simulink model "RPL_3D_Mode_BlocksetApproach"  (R2021b)
settings: Solver=VariableStepAuto  StartTime=0.0  StopTime=10.0  RelTol=1e-3
values from neighbouring files (symbols this model uses):
  Ar = pi*R_rad^2    (= 0.00282743338823)    [constants1DoF.m]
  Cd = 0.5    [constants1DoF.m]
  g = 9.81    [constants1DoF.m]
  m_d_c = 0.01    [constants1DoF.m]
  m_r = 0.5    [constants1DoF.m]
  rho = 1.225    [constants1DoF.m]
  t_burn = 2    [constants1DoF.m]
  Tmax = 10    [constants1DoF.m]
libraries: aerolibbdyn x2, sharedutil x1, aerolibanim x1, aerolib6dof2 x1
settings Model: Creator=josep  LastModifiedBy=josepfamador

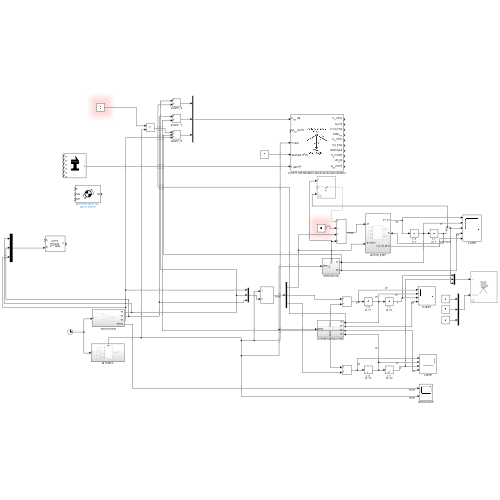
[thumbnail: Simulink's stored preview of the top-level diagram]
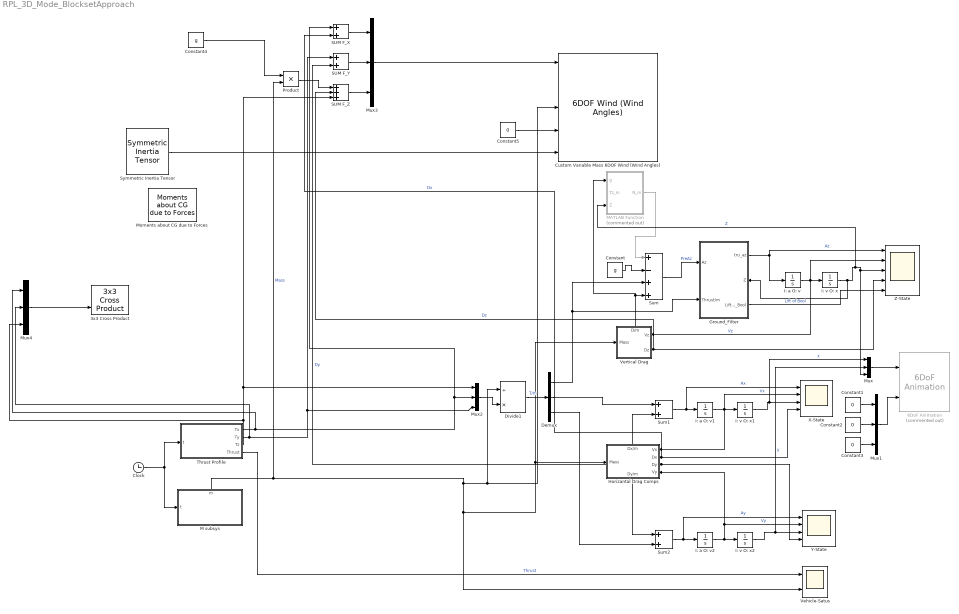
== system RPL_3D_Mode_BlocksetApproach ==
  3x3 Cross Product : sharedutil/3x3 Cross Product  aMode=aMode
      settings: SourceProductBaseCode=AE,PW,DR,MT,UV,VE
  6DoF Animation : aerolibanim/6DoF Animation  Commented=on  u1=[-400 400 -200 200 -500 -300]  u2=0.1  u3=10.0  u4=[0 0 0]  u5=Cockpit  u6=[100 50 -50]  u7=10  u8=on
  Clock : Clock
      settings: Decimation=5
  Constant : Constant  Value=g
  Constant{1..3,5} (4 alike) : Constant  Value=0
  Constant4 : Constant  Value=g
  Custom Variable Mass 6DOF Wind (Wind Angles) : aerolib6dof2/6DOF Wind (Wind Angles)  units=Metric (MKS)  mtype=Custom Variable  rep=Wind Angles  xme_0=[0 0 0]  Vm_0=[0 0 0]  wind_0=[0 0 0]  pm_0=[0 0 0]  mass_0=1.0  mass_e=0.5  mass_f=2.0  inertia=eye(3)  inertia_e=eye(3)  inertia_f=2*eye(3)  vre_flag=off  abi_flag=off  xme_statename=''  Vm_statename=''  alpha_statename=''  beta_statename=''  wind_statename=''  quat_statename=''  pm_statename=''  mass_statename=''
      settings: SourceProductBaseCode=AE
  Demux : Demux  Outputs=3
  Divide1 : Product  Inputs=/*
  Ground_Filter : Subsystem
      settings: PortSchema="{\"entries\":[{\"content\":{\"sides\":[{\"content\":{\"connectorIds\":[\"In1\",\"In2\"]},\"type\":\"ConnectorPlacement.EquallySpacedRectSide\",\"uuid\":\"02f139e3-c71d-4215-a05c-2ea7cb935f0c\"},{\"content\":{\"connectorIds\":[\"Out1\",\"In3\",\"Out2\"],\"side\":\"RIGHT\"},\"type\":\"ConnectorPlacement.EquallySpacedRectSide\",\"uuid\":\"f8d88dc7-1706-414e-8763-66b2344e60f3\"},{\"content\":{\"connectorIds\":[],\"side\":\"TOP\"},\"type\":\"ConnectorPlacement.EquallySpacedRectSide\",\"uuid\":\"2e6fab3d-690f-4ad2-8e7d-0c65fcb07007\"}]},\"type\":\"ConnectorPlacement.EquallySpacedConnector\",\"uuid\":\"04f6aaf0-68c8-473c-8854-b1e33576e060\"}],\"packageUris\":[\"http://schema.mathworks.com/mf0/Connector/R2020b\"],\"version\":\"1.0\"}"
  Horizantal Drag Comps : Subsystem
      settings: PortSchema="{\"entries\":[{\"content\":{\"sides\":[{\"content\":{\"connectorIds\":[\"In1\"]},\"type\":\"ConnectorPlacement.EquallySpacedRectSide\",\"uuid\":\"a9ae7cae-0740-4af7-9b70-c16e835fd7b3\"},{\"content\":{\"connectorIds\":[\"In2\",\"Out1\",\"Out2\",\"In3\"],\"side\":\"RIGHT\"},\"type\":\"ConnectorPlacement.EquallySpacedRectSide\",\"uuid\":\"8697e8bb-b6ea-43ee-b298-40652abd00a9\"},{\"content\":{\"connectorIds\":[\"Out4\"],\"side\":\"TOP\"},\"type\":\"ConnectorPlacement.EquallySpacedRectSide\",\"uuid\":\"6019ad8c-fb7f-40d5-87eb-98a170a5ecc9\"},{\"content\":{\"connectorIds\":[\"Out3\"],\"side\":\"BOTTOM\"},\"type\":\"ConnectorPlacement.EquallySpacedRectSide\",\"uuid\":\"b4d29286-deca-444a-b294-c191927f4c5c\"}]},\"type\":\"ConnectorPlacement.EquallySpacedConnector\",\"uuid\":\"482fa5f4-cfef-448e-9d08-7fbc847693c8\"}],\"packageUris\":[\"http://schema.mathworks.com/mf0/Connector/R2020b\"],\"version\":\"1.0\"}"
  I: a O: v : Integrator
  I: a O: v1 : Integrator
  I: a O: v2 : Integrator
  I: v O: x : Integrator  LowerSaturationLimit=0
  I: v O: x1 : Integrator  LowerSaturationLimit=0
  I: v O: x2 : Integrator  LowerSaturationLimit=0
  M subsys : Subsystem
      settings: PortSchema="{\"entries\":[{\"content\":{\"sides\":[{\"content\":{\"connectorIds\":[\"In1\"]},\"type\":\"ConnectorPlacement.EquallySpacedRectSide\",\"uuid\":\"59fe94dd-ab30-4deb-857c-de4b730c9c49\"},{\"content\":{\"connectorIds\":[],\"side\":\"RIGHT\"},\"type\":\"ConnectorPlacement.EquallySpacedRectSide\",\"uuid\":\"6db86113-106d-42a4-8531-3673608ca4b9\"},{\"content\":{\"connectorIds\":[\"Out1\"],\"side\":\"TOP\"},\"type\":\"ConnectorPlacement.EquallySpacedRectSide\",\"uuid\":\"45854090-be75-4cdf-9468-5c433929868a\"}]},\"type\":\"ConnectorPlacement.EquallySpacedConnector\",\"uuid\":\"b924312b-0fe7-4021-be64-7e2ca8cc4ab7\"}],\"packageUris\":[\"http://schema.mathworks.com/mf0/Connector/R2020b\"],\"version\":\"1.0\"}"
  MATLAB Function : MATLAB Function  Commented=on  TreatAsAtomicUnit=on
  Moments about CG due to Forces : aerolibbdyn/Moments about CG  due to Forces
      settings: SourceProductBaseCode=AE
  Mux{,1..4} (5 alike) : Mux  Inputs=3
  Product : Product
  SUM F_X : Sum
  SUM F_Y : Sum
  SUM F_Z : Sum  Inputs=+++
  Sum : Sum  Inputs=+-++
  Sum1 : Sum
  Sum2 : Sum
  Symmetric Inertia Tensor : aerolibbdyn/Symmetric Inertia Tensor
      settings: SourceProductBaseCode=AE
  Thrust Profile : Subsystem
  Vehicle-Satus : Scope  NumInputPorts=2
  Vertical Drag : Subsystem
      settings: PortSchema="{\"entries\":[{\"content\":{\"sides\":[{\"content\":{\"connectorIds\":[\"In1\"]},\"type\":\"ConnectorPlacement.EquallySpacedRectSide\",\"uuid\":\"72cb64b5-de92-49f0-81ee-1566d770d166\"},{\"content\":{\"connectorIds\":[\"In2\",\"Out1\"],\"side\":\"RIGHT\"},\"type\":\"ConnectorPlacement.EquallySpacedRectSide\",\"uuid\":\"ba77af52-770b-4a76-8b2e-e7cb196d7331\"},{\"content\":{\"connectorIds\":[\"Out2\"],\"side\":\"TOP\"},\"type\":\"ConnectorPlacement.EquallySpacedRectSide\",\"uuid\":\"b46aeb0c-d0a3-4548-b994-998d7dcb34ee\"}]},\"type\":\"ConnectorPlacement.EquallySpacedConnector\",\"uuid\":\"4a9965ec-71ae-4d95-8721-5a5c59972a5c\"}],\"packageUris\":[\"http://schema.mathworks.com/mf0/Connector/R2020b\"],\"version\":\"1.0\"}"
  X-State : Scope  NumInputPorts=4
  Y-State : Scope  NumInputPorts=4
  Z-State : Scope  NumInputPorts=5
  wires:
  Horizantal Drag Comps/4(Dx/m) -> Sum1/2
  Thrust Profile/1(Tx) -> Mux4/1, Mux2/2, SUM F_X/1
  Ground_Filter/2(Lift_off_Bool) -> Z-State/5  "Lift of Bool"
  Vertical Drag/2(D/m) -> MATLAB Function/1(g), Sum/4
  MATLAB Function/1(N_m) -> Sum/1
  Sum/1 -> Ground_Filter/1(Az)  "PreAz"
  Horizantal Drag Comps/2(Dy) -> Y-State/4, SUM F_Y/2  "Dy"
  Sum1/1 -> X-State/1, I: a O: v1/1  "Ax"
  Thrust Profile/2(Ty) -> Mux4/2, SUM F_Y/1, Mux2/3
  Vertical Drag/1(Dz) -> Z-State/4, SUM F_Z/2  "Dz"
  M subsys/1(m) -> Custom Variable Mass 6DOF Wind (Wind Angles)/3, Divide1/1, Vehicle-Satus/2, Vertical Drag/1(Mass), Horizantal Drag Comps/1(Mass), Product/2  "Mass"
  Thrust Profile/3(Tz) -> Mux4/3, SUM F_Z/3, Mux2/1
  Horizantal Drag Comps/1(Dx) -> X-State/4, SUM F_X/2  "Dx"
  Constant3/1 -> Mux1/3
  Ground_Filter/1(tru_az) -> I: a O: v/1, Z-State/1  "Az"
  Constant/1 -> Sum/2
  Constant1/1 -> Mux1/1
  I: a O: v/1 -> Vertical Drag/2(Vz), Z-State/2, I: v O: x/1  "Vz"
  Mux/1 -> 6DoF Animation/1
  Constant2/1 -> Mux1/2
  I: v O: x/1 -> Ground_Filter/3(Z), MATLAB Function/3(Z), Mux/3, Z-State/3  "Z"
  I: a O: v2/1 -> Horizantal Drag Comps/3(Vy), Y-State/2, I: v O: x2/1  "Vy"
  Mux1/1 -> 6DoF Animation/2
  I: v O: x2/1 -> Mux/2, Y-State/3  "y"
  Horizantal Drag Comps/3(Dy/m) -> Sum2/1
  Clock/1 -> M subsys/1(t), Thrust Profile/1(t)
  Thrust Profile/4(Thrust) -> Vehicle-Satus/1  "Thrust"
  I: v O: x1/1 -> Mux/1, X-State/3  "x"
  Sum2/1 -> Y-State/1, I: a O: v2/1  "Ay"
  I: a O: v1/1 -> X-State/2, Horizantal Drag Comps/2(Vx), I: v O: x1/1  "Vx"
  Constant4/1 -> Product/1
  Product/1 -> SUM F_Z/1
  Mux2/1 -> Divide1/2
  Divide1/1 -> Demux/1  "T/m"
  Demux/1 -> Ground_Filter/2(Thrust/m), Sum/3
  Demux/2 -> Sum1/1
  Demux/3 -> Sum2/2
  SUM F_Z/1 -> Mux3/3
  SUM F_Y/1 -> Mux3/2
  SUM F_X/1 -> Mux3/1
  Mux3/1 -> Custom Variable Mass 6DOF Wind (Wind Angles)/1
  Constant5/1 -> Custom Variable Mass 6DOF Wind (Wind Angles)/4
  Symmetric Inertia Tensor/1 -> Custom Variable Mass 6DOF Wind (Wind Angles)/5
  Mux4/1 -> 3x3 Cross Product/2

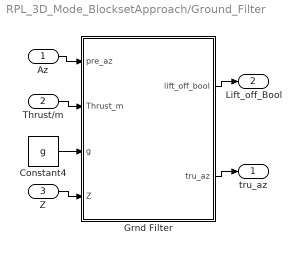
== system RPL_3D_Mode_BlocksetApproach/Ground_Filter ==
  Az : Inport
  Thrust/m : Inport  Port=2
  Z : Inport  Port=3
  Constant4 : Constant  Value=g
  Grnd Filter : MATLAB Function  TreatAsAtomicUnit=on
  tru_az : Outport
  Lift_off_Bool : Outport  Port=2
  wires:
  Constant4/1 -> Grnd Filter/3(g)
  Az/1 -> Grnd Filter/1(pre_az)
  Thrust/m/1 -> Grnd Filter/2(Thrust_m)
  Grnd Filter/2(tru_az) -> tru_az/1
  Grnd Filter/1(lift_off_bool) -> Lift_off_Bool/1
  Z/1 -> Grnd Filter/4(Z)

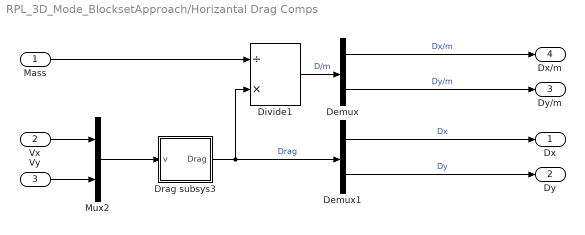
== system RPL_3D_Mode_BlocksetApproach/Horizantal Drag Comps ==
  Mass : Inport
  Vx : Inport  Port=2
  Vy : Inport  Port=3
  Demux : Demux  Outputs=2
  Demux1 : Demux  Outputs=2
  Divide1 : Product  Inputs=/*
  Drag subsys3 : Subsystem
      settings: PortSchema="{\"entries\":[{\"content\":{\"sides\":[{\"content\":{\"connectorIds\":[\"Out1\"]},\"type\":\"ConnectorPlacement.EquallySpacedRectSide\",\"uuid\":\"59fe94dd-ab30-4deb-857c-de4b730c9c49\"},{\"content\":{\"connectorIds\":[\"In1\"],\"side\":\"RIGHT\"},\"type\":\"ConnectorPlacement.EquallySpacedRectSide\",\"uuid\":\"6db86113-106d-42a4-8531-3673608ca4b9\"},{\"content\":{\"connectorIds\":[],\"side\":\"TOP\"},\"type\":\"ConnectorPlacement.EquallySpacedRectSide\",\"uuid\":\"45854090-be75-4cdf-9468-5c433929868a\"}]},\"type\":\"ConnectorPlacement.EquallySpacedConnector\",\"uuid\":\"b924312b-0fe7-4021-be64-7e2ca8cc4ab7\"}],\"packageUris\":[\"http://schema.mathworks.com/mf0/Connector/R2020b\"],\"version\":\"1.0\"}"
  Mux2 : Mux  Inputs=2
  Dx : Outport
  Dy : Outport  Port=2
  Dy/m : Outport  Port=3
  Dx/m : Outport  Port=4
  wires:
  Drag subsys3/1(Drag) -> Divide1/2, Demux1/1  "Drag"
  Divide1/1 -> Demux/1  "D/m"
  Mux2/1 -> Drag subsys3/1(v)
  Vy/1 -> Mux2/2
  Demux1/1 -> Dx/1  "Dx"
  Demux1/2 -> Dy/1  "Dy"
  Vx/1 -> Mux2/1
  Demux/2 -> Dy/m/1  "Dy/m"
  Demux/1 -> Dx/m/1  "Dx/m"
  Mass/1 -> Divide1/1

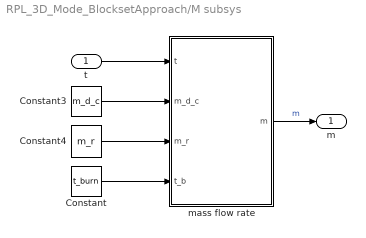
== system RPL_3D_Mode_BlocksetApproach/M subsys ==
  t : Inport
  Constant : Constant  Value=t_burn
  Constant3 : Constant  Value=m_d_c
  Constant4 : Constant  Value=m_r
  mass flow rate : MATLAB Function  TreatAsAtomicUnit=on
  m : Outport
  wires:
  t/1 -> mass flow rate/1(t)
  Constant3/1 -> mass flow rate/2(m_d_c)
  Constant4/1 -> mass flow rate/3(m_r)
  mass flow rate/1(m) -> m/1  "m"
  Constant/1 -> mass flow rate/4(t_b)

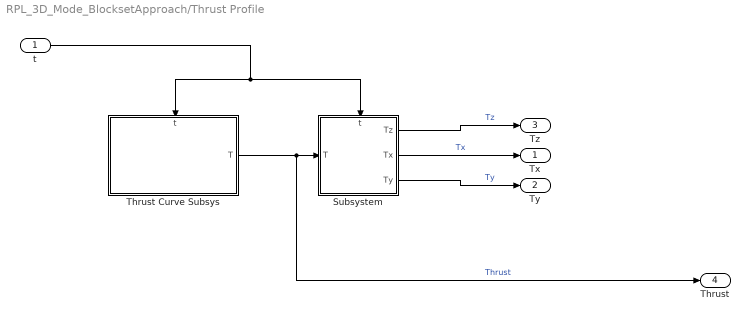
== system RPL_3D_Mode_BlocksetApproach/Thrust Profile ==
  t : Inport
  Subsystem : Subsystem
      settings: PortSchema="{\"entries\":[{\"content\":{\"sides\":[{\"content\":{\"connectorIds\":[\"In1\"]},\"type\":\"ConnectorPlacement.EquallySpacedRectSide\",\"uuid\":\"018992c4-8275-41b6-b967-28a58c9ca20f\"},{\"content\":{\"connectorIds\":[\"Out1\",\"Out2\",\"Out3\"],\"side\":\"RIGHT\"},\"type\":\"ConnectorPlacement.EquallySpacedRectSide\",\"uuid\":\"629673e7-0247-4186-892d-9522b2c54d6d\"},{\"content\":{\"connectorIds\":[\"In2\"],\"side\":\"TOP\"},\"type\":\"ConnectorPlacement.EquallySpacedRectSide\",\"uuid\":\"a618db3c-6ebf-4698-8fd3-162c3d081110\"}]},\"type\":\"ConnectorPlacement.EquallySpacedConnector\",\"uuid\":\"c7f983df-0e64-40e7-bc45-4793f07a667f\"}],\"packageUris\":[\"http://schema.mathworks.com/mf0/Connector/R2020b\"],\"version\":\"1.0\"}"
  Thrust Curve Subsys : Subsystem
      settings: PortSchema="{\"entries\":[{\"content\":{\"sides\":[{\"content\":{\"connectorIds\":[]},\"type\":\"ConnectorPlacement.EquallySpacedRectSide\",\"uuid\":\"59fe94dd-ab30-4deb-857c-de4b730c9c49\"},{\"content\":{\"connectorIds\":[\"Out1\"],\"side\":\"RIGHT\"},\"type\":\"ConnectorPlacement.EquallySpacedRectSide\",\"uuid\":\"6db86113-106d-42a4-8531-3673608ca4b9\"},{\"content\":{\"connectorIds\":[\"In1\"],\"side\":\"TOP\"},\"type\":\"ConnectorPlacement.EquallySpacedRectSide\",\"uuid\":\"45854090-be75-4cdf-9468-5c433929868a\"}]},\"type\":\"ConnectorPlacement.EquallySpacedConnector\",\"uuid\":\"b924312b-0fe7-4021-be64-7e2ca8cc4ab7\"}],\"packageUris\":[\"http://schema.mathworks.com/mf0/Connector/R2020b\"],\"version\":\"1.0\"}"
  Tx : Outport
  Ty : Outport  Port=2
  Tz : Outport  Port=3
  Thrust : Outport  Port=4
  wires:
  Thrust Curve Subsys/1(T) -> Thrust/1, Subsystem/1(T)  "Thrust"
  Subsystem/2(Tx) -> Tx/1  "Tx"
  Subsystem/3(Ty) -> Ty/1  "Ty"
  Subsystem/1(Tz) -> Tz/1  "Tz"
  t/1 -> Subsystem/2(t), Thrust Curve Subsys/1(t)

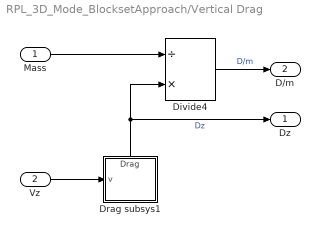
== system RPL_3D_Mode_BlocksetApproach/Vertical Drag ==
  Mass : Inport
  Vz : Inport  Port=2
  Divide4 : Product  Inputs=/*
  Drag subsys1 : Subsystem
      settings: PortSchema="{\"entries\":[{\"content\":{\"sides\":[{\"content\":{\"connectorIds\":[]},\"type\":\"ConnectorPlacement.EquallySpacedRectSide\",\"uuid\":\"59fe94dd-ab30-4deb-857c-de4b730c9c49\"},{\"content\":{\"connectorIds\":[\"In1\"],\"side\":\"RIGHT\"},\"type\":\"ConnectorPlacement.EquallySpacedRectSide\",\"uuid\":\"6db86113-106d-42a4-8531-3673608ca4b9\"},{\"content\":{\"connectorIds\":[],\"side\":\"TOP\"},\"type\":\"ConnectorPlacement.EquallySpacedRectSide\",\"uuid\":\"45854090-be75-4cdf-9468-5c433929868a\"},{\"content\":{\"connectorIds\":[\"Out1\"],\"side\":\"BOTTOM\"},\"type\":\"ConnectorPlacement.EquallySpacedRectSide\",\"uuid\":\"cf9973e3-0315-4fb8-9650-314bde500f3f\"}]},\"type\":\"ConnectorPlacement.EquallySpacedConnector\",\"uuid\":\"b924312b-0fe7-4021-be64-7e2ca8cc4ab7\"}],\"packageUris\":[\"http://schema.mathworks.com/mf0/Connector/R2020b\"],\"version\":\"1.0\"}"
  Dz : Outport
  D/m : Outport  Port=2
  wires:
  Vz/1 -> Drag subsys1/1(v)
  Mass/1 -> Divide4/1
  Divide4/1 -> D/m/1  "D/m"
  Drag subsys1/1(Drag) -> Dz/1, Divide4/2  "Dz"

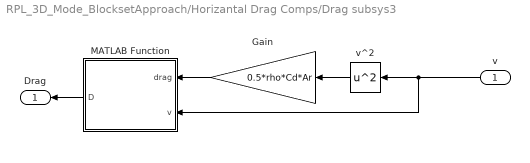
== system RPL_3D_Mode_BlocksetApproach/Horizantal Drag Comps/Drag subsys3 ==
  v : Inport
  Gain : Gain  Gain=0.5*rho*Cd*Ar
  MATLAB Function : MATLAB Function  TreatAsAtomicUnit=on
  v^2 : Math  Operator=square  SaturateOnIntegerOverflow=on
  Drag : Outport
  wires:
  v^2/1 -> Gain/1
  Gain/1 -> MATLAB Function/1(drag)
  MATLAB Function/1(D) -> Drag/1
  v/1 -> MATLAB Function/2(v), v^2/1

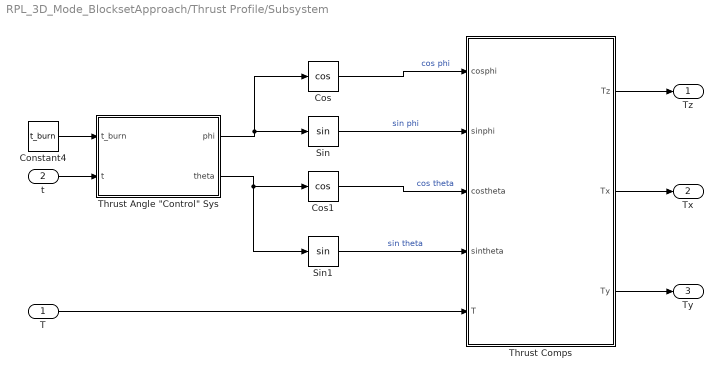
== system RPL_3D_Mode_BlocksetApproach/Thrust Profile/Subsystem ==
  T : Inport
  t : Inport  Port=2
  Constant4 : Constant  Value=t_burn
  Cos : Trigonometry  Operator=cos
  Cos1 : Trigonometry  Operator=cos
  Sin : Trigonometry
  Sin1 : Trigonometry
  "Thrust Angle \"Control\" Sys" : MATLAB Function  TreatAsAtomicUnit=on
  Thrust Comps : MATLAB Function  TreatAsAtomicUnit=on
  Tz : Outport
  Tx : Outport  Port=2
  Ty : Outport  Port=3
  wires:
  Cos1/1 -> Thrust Comps/3(costheta)  "cos theta"
  "Thrust Angle \"Control\" Sys"/2(theta) -> Sin1/1, Cos1/1
  "Thrust Angle \"Control\" Sys"/1(phi) -> Sin/1, Cos/1
  Sin1/1 -> Thrust Comps/4(sintheta)  "sin theta"
  Constant4/1 -> "Thrust Angle \"Control\" Sys"/1(t_burn)
  t/1 -> "Thrust Angle \"Control\" Sys"/2(t)
  Cos/1 -> Thrust Comps/1(cosphi)  "cos phi"
  Sin/1 -> Thrust Comps/2(sinphi)  "sin phi"
  T/1 -> Thrust Comps/5(T)
  Thrust Comps/1(Tz) -> Tz/1
  Thrust Comps/2(Tx) -> Tx/1
  Thrust Comps/3(Ty) -> Ty/1

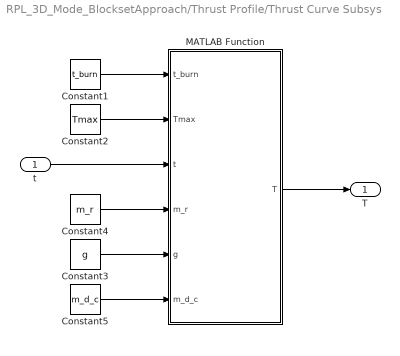
== system RPL_3D_Mode_BlocksetApproach/Thrust Profile/Thrust Curve Subsys ==
  t : Inport
  Constant1 : Constant  Value=t_burn
  Constant2 : Constant  Value=Tmax
  Constant3 : Constant  Value=g
  Constant4 : Constant  Value=m_r
  Constant5 : Constant  Value=m_d_c
  MATLAB Function : MATLAB Function  TreatAsAtomicUnit=on
  T : Outport
  wires:
  Constant1/1 -> MATLAB Function/1(t_burn)
  Constant2/1 -> MATLAB Function/2(Tmax)
  t/1 -> MATLAB Function/3(t)
  MATLAB Function/1(T) -> T/1
  Constant3/1 -> MATLAB Function/5(g)
  Constant4/1 -> MATLAB Function/4(m_r)
  Constant5/1 -> MATLAB Function/6(m_d_c)

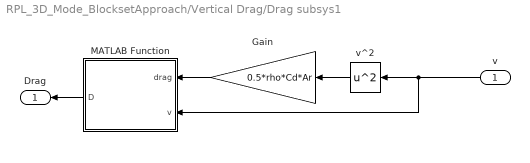
== system RPL_3D_Mode_BlocksetApproach/Vertical Drag/Drag subsys1 ==
  v : Inport
  Gain : Gain  Gain=0.5*rho*Cd*Ar
  MATLAB Function : MATLAB Function  TreatAsAtomicUnit=on
  v^2 : Math  Operator=square  SaturateOnIntegerOverflow=on
  Drag : Outport
  wires:
  v^2/1 -> Gain/1
  Gain/1 -> MATLAB Function/1(drag)
  MATLAB Function/1(D) -> Drag/1
  v/1 -> MATLAB Function/2(v), v^2/1

== matlab function RPL_3D_Mode_BlocksetApproach/M subsys/mass flow rate ==
  data: t input; m output; m_d_c input; m_r input; t_b input
function m = m_flow(t, m_d_c, m_r, t_b)
%Const Define in 'constants1DoF.m'
%out mass at time t


if t <= t_b 
    m= -m_d_c*t + m_r;
else
    m = -m_d_c*t_b + m_r;
end

== matlab function RPL_3D_Mode_BlocksetApproach/Thrust Profile/Thrust Curve Subsys/MATLAB Function ==
  data: t_burn input; Tmax input; t input; m_r input; T output; g input; m_d_c input
function T = T_of_t(t_burn, Tmax, t, m_r, g,m_d_c)
%Approx Thurst Curve.
%Total Burn time = 1s
%Max Thrust 100N

%Constants Defined in 'constants1DoF.m'
x_hf = t_burn/2;
a = Tmax/((x_hf)*(x_hf - t_burn));

%linear down slope after peak thrust

%Consider making weight dynamic function later
w_f = m_r*g - t_burn*m_d_c; %Final Weight

slope = (w_f - Tmax)/(0.5*t_burn);

if t<=0
    T = 0; %ded

elseif t<t_burn*0.5
    T = a*t*(t-t_burn); %lift off burn

elseif t<=t_burn
    T = slope * (t - t_burn*0.5) + Tmax;
else
    %T = w_f;
    T = 0; 
end

== matlab function RPL_3D_Mode_BlocksetApproach/Vertical Drag/Drag subsys1/MATLAB Function ==
  data: drag input; D output; v input
function D = sign_change(drag, v)
%changes signs of Drag when appropiate. Drag is always opposite to velocity

if v>0
    D = -drag;
else
    D = drag;
end

== matlab function RPL_3D_Mode_BlocksetApproach/MATLAB Function ==
  data: g input; N_m output; Tz_m input; Z input
function N_m = fcn(g , Tz_m, Z)

if Z <= 0
    N_m = g - Tz_m;
else
    N_m = 0;
end

== matlab function RPL_3D_Mode_BlocksetApproach/Thrust Profile/Subsystem/Thrust Angle "Control" Sys ==
  data: t_burn input; t input; phi output; theta output
function [phi,theta] = T_angle(t_burn, t)
%Assuming Spherical Coordinates
dummyconst = 1; %random debug/test const.

if t<=t_burn
    theta = 0;
    phi = 0;
else
    theta = dummyconst * t;
    phi = pi/2;
end

== matlab function RPL_3D_Mode_BlocksetApproach/Horizantal Drag Comps/Drag subsys3/MATLAB Function ==
  data: drag input; D output; v input
function D = sign_change(drag, v)
%changes signs of Drag when appropiate. Drag is always opposite to velocity

if v>0
    D = -drag;
else
    D = drag;
end

== matlab function RPL_3D_Mode_BlocksetApproach/Ground_Filter/Grnd Filter ==
  data: lift_off_bool output; pre_az input; tru_az output; Thrust_m input; g input; Z input
function [lift_off_bool, tru_az]= grndFilter(pre_az, Thrust_m, g, Z)
%Ground condition. Acc = 0 until Thrust > weight

if Thrust_m<=g && Z==0
    lift_off_bool = false;
    tru_az = 0;
else
    tru_az = pre_az;
    lift_off_bool = true;
end

== matlab function RPL_3D_Mode_BlocksetApproach/Thrust Profile/Subsystem/Thrust Comps ==
  data: Tz output; cosphi input; Tx output; sinphi input; costheta input; sintheta input; T input; Ty output
function [Tz, Tx, Ty] = fcn(cosphi,sinphi,costheta,sintheta, T)

Txy = T*sinphi; %T Proj onto xy-plane

Tz = T*cosphi;
Tx = Txy*costheta;
Ty = Txy*sintheta;
end
